simulink model "Master_PD_Operator"  (R2020a)
settings: Solver=VariableStepAuto  StartTime=0.0  StopTime=10  RelTol=1e-3
values from neighbouring files (symbols this model uses):
  Bh = 0.02    [Teleop_parameters.m]    (also in base.mat; base_no_attrito.mat; ci_siamo.mat; force_control.mat)
  Jh = 0.02    [Teleop_parameters.m]    (also in base.mat; base_no_attrito.mat; ci_siamo.mat; force_control.mat)
  k_m = 19.34    [Teleop_parameters.m]    (also in base.mat; base_no_attrito.mat; ci_siamo.mat; force_control.mat)
  Kc2v_m = 2    [Teleop_parameters.m]    (also in base.mat; base_no_attrito.mat; ci_siamo.mat; force_control.mat)
  Kt2c_m = 1.182    [Teleop_parameters.m]    (also in base.mat; base_no_attrito.mat; ci_siamo.mat; force_control.mat)
  lArm_m = 0.1    [Teleop_parameters.m]    (also in base.mat; base_no_attrito.mat; ci_siamo.mat; force_control.mat)
  maxCurrent_m = 4.5    [Teleop_parameters.m]    (also in base.mat; base_no_attrito.mat; ci_siamo.mat; force_control.mat)
  tau_m = 1.217    [Teleop_parameters.m]    (also in base.mat; base_no_attrito.mat; ci_siamo.mat; force_control.mat)
settings Model: Creator=riccardo  LastModifiedBy=gbagolin

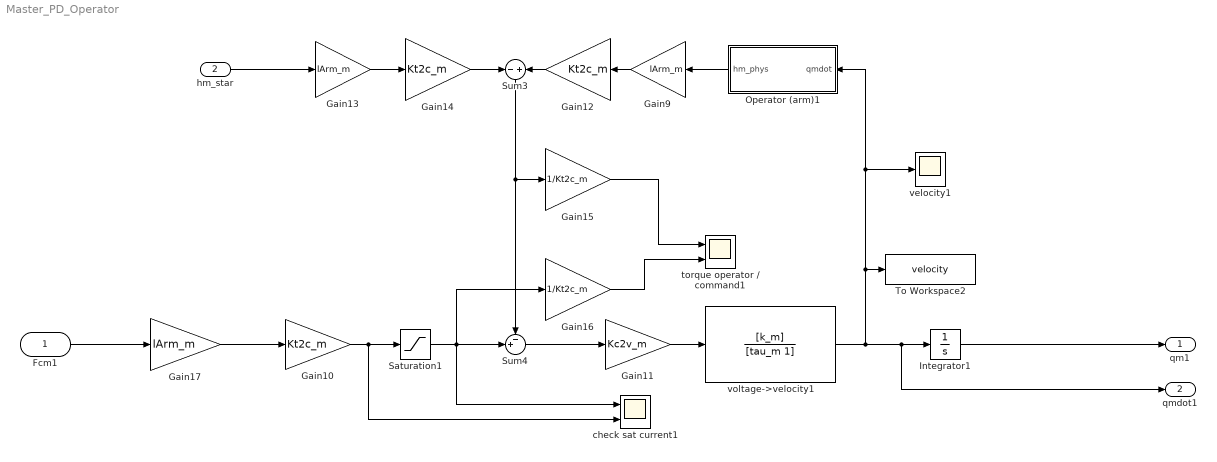
== system Master_PD_Operator ==
  Fcm1 : Inport
  hm_star : Inport  Port=2
  Gain10 : Gain  Gain=Kt2c_m
  Gain11 : Gain  Gain=Kc2v_m
  Gain12 : Gain  Gain=Kt2c_m
  Gain13 : Gain  Gain=lArm_m
  Gain14 : Gain  Gain=Kt2c_m
  Gain15 : Gain  Gain=1/Kt2c_m
  Gain16 : Gain  Gain=1/Kt2c_m
  Gain17 : Gain  Gain=lArm_m
  Gain9 : Gain  Gain=lArm_m
  Integrator1 : Integrator
  Operator (arm)1 : Subsystem
  Saturation1 : Saturate  UpperLimit=maxCurrent_m  LowerLimit=-maxCurrent_m
  Sum3 : Sum  Inputs=-+
  Sum4 : Sum  Inputs=-+|
  To Workspace2 : ToWorkspace  VariableName=velocity  SaveFormat=Timeseries  SampleTime=-1
  check sat current1 : Scope  NumInputPorts=2
  torque operator / command1 : Scope  NumInputPorts=2
  velocity1 : Scope
  voltage->velocity1 : TransferFcn  Numerator=[k_m]  Denominator=[tau_m 1]
  qm1 : Outport
  qmdot1 : Outport  Port=2
  wires:
  Gain17/1 -> Gain10/1
  voltage->velocity1/1 -> velocity1/1, Operator (arm)1/1(qmdot), To Workspace2/1, qmdot1/1, Integrator1/1
  Sum3/1 -> Sum4/1, Gain15/1
  Integrator1/1 -> qm1/1
  Gain12/1 -> Sum3/2
  Gain16/1 -> torque operator / command1/2
  Gain11/1 -> voltage->velocity1/1
  Saturation1/1 -> Gain16/1, Sum4/2, check sat current1/1
  Gain14/1 -> Sum3/1
  Gain15/1 -> torque operator / command1/1
  Operator (arm)1/1(hm_phys) -> Gain9/1
  Gain9/1 -> Gain12/1
  Fcm1/1 -> Gain17/1
  Gain13/1 -> Gain14/1
  Sum4/1 -> Gain11/1
  Gain10/1 -> check sat current1/2, Saturation1/1
  hm_star/1 -> Gain13/1

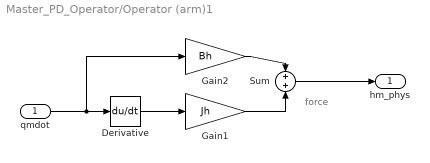
== system Master_PD_Operator/Operator (arm)1 ==
  note: force
  qmdot : Inport
  Derivative : Derivative  CoefficientInTFapproximation=0.001
  Gain1 : Gain  Gain=Jh
  Gain2 : Gain  Gain=Bh
  Sum : Sum  Inputs=+|+
  hm_phys : Outport  VectorParamsAs1DForOutWhenUnconnected=off
  wires:
  qmdot/1 -> Gain2/1, Derivative/1
  Sum/1 -> hm_phys/1
  Derivative/1 -> Gain1/1
  Gain2/1 -> Sum/1
  Gain1/1 -> Sum/2
